simulink model "canal_dynamics"  (Simulink 7.1)
settings: Solver=ode45  StartTime=0.0  StopTime=10.0  FixedStep=1  RelTol=1e-3
values from neighbouring files (symbols this model uses):
  T = 0.015    [canal_afferent_step_response.m]
  T1 = 5.7    [canal_afferent_step_response.m]
  T2 = 0.003    [canal_afferent_step_response.m]
  Ts = simoutTP    [canal_afferent_step_response.m]
settings Model: Creator=adams  LastModifiedBy=adams
settings DebuggingCC: SaveWithParameterizedLinksMsg=none  SignalResolutionControl=TryResolveAllWithWarning  MultiTaskDSMMsg=warning  MultiTaskCondExecSysMsg=none  StrictBusMsg=None
settings RTWCC: IncludeERTFirstTime=on
settings GRTTargetCC: TargetFcnLib=ansi_tfl_tmw.mat

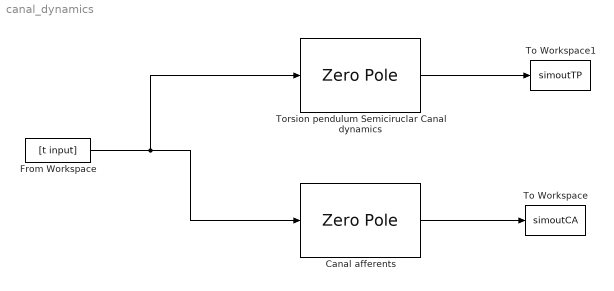
== system canal_dynamics ==
  "Canal afferents " : ZeroPole  Zeros=[0 -1/T]  Poles=[-1/T1 -1/T2]  Gain=[T/(T1*T2)]
  From Workspace : FromWorkspace  VariableName=[t input]  SampleTime=Ts
  To Workspace : ToWorkspace  VariableName=simoutCA  SampleTime=Ts  SaveFormat=Array
  To Workspace1 : ToWorkspace  VariableName=simoutTP  SampleTime=Ts  SaveFormat=Array
  Torsion pendulum Semiciruclar Canal dynamics : ZeroPole  Zeros=[]  Poles=[-1/T1 -1/T2]  Gain=[1/(T1*T2)]
  wires:
  From Workspace/1 -> "Canal afferents "/1, Torsion pendulum Semiciruclar Canal dynamics/1
  "Canal afferents "/1 -> To Workspace/1
  Torsion pendulum Semiciruclar Canal dynamics/1 -> To Workspace1/1
